simulink model "Simulation_Fahrmodell_v4_straight_line_v2"  (R2023b)
settings: Solver=ode14x  StartTime=0.0  StopTime=500  FixedStep=0.005  RelTol=1e-3
undefined symbols (not defined in the file): bat, cp, cp_Zelle_JpkgK, gb, gb_Gear_Ratio_LUT, gb_Gears_LUT, Ice_derfacLoadDecrease_MAP, Ice_derfacLoadIncrease_MAP, Ice_n_axis, Ice_relLoadMax_CUR_n, Ice_relLoadMax_CUR_val, Ice_rl_axis_norm, P4, P4_DM, pt, seconds, SKO_STREET_CHAL, SKO_WHEEL_TYP_CHAL, slip_pacejka, T_init_degC, Track, TT_sliced, use_turbo_model, v_Fzg_init_kmph, veh, vmax_driver_target_kmh
libraries: nesl_utility x15, fl_lib x9, simulink x4
(part 7 of 7)

== matlab function Simulation_Fahrmodell_v4_straight_line_v2/Vehicle Dynamics Model /Drivetrain/Primary and Secondary Axle Powertrain Selector/MATLAB Function2 ==
  data: Tq_in input; Tq_out output; launchFactor input
function Tq_out = apply_launch_factor(Tq_in, launchFactor)
%#codegen

if Tq_in > 0
    Tq_out = Tq_in * launchFactor;
else
    Tq_out = Tq_in;
end
end

== matlab function Simulation_Fahrmodell_v4_straight_line_v2/Vehicle Dynamics Model /Drivetrain/Axle Load and Torque Distribution /Berechnung Achslastverteilung abh. Fahrzeugeigenschaften (Haken Abs. 11)/MATLAB Function ==
  data: u input; y output
function y = cosd(u)

y = cosd(u);

== matlab function Simulation_Fahrmodell_v4_straight_line_v2/Vehicle Dynamics Model /Drivetrain/Axle Load and Torque Distribution /Berechnung Achslastverteilung abh. Fahrzeugeigenschaften (Haken Abs. 11)/MATLAB Function1 ==
  data: u input; y output
function y = sind(u)

y = sind(u);

== matlab function Simulation_Fahrmodell_v4_straight_line_v2/Vehicle Dynamics Model /Drivetrain/Operating Strategy 1.1/Axle Torque Split/MATLAB Function1 ==
  data: P4_deactivate output; Torque_ICE_Axle_percent output; SOC input; cfg_P4 input; EV input; MainAxle_TorqueSplit_int input; Torque_P4_Axle_percent output
function [P4_deactivate, Torque_ICE_Axle_percent, Torque_P4_Axle_percent]...
        = TorqueSplit(SOC, cfg_P4, EV, MainAxle_TorqueSplit_int)

    % State memory for hysteresis (Lockout flag)
    persistent p4_low_soc_lockout
    if isempty(p4_low_soc_lockout)
        p4_low_soc_lockout = false; 
    end

    % Default: ICE takes all torque, P4 takes none
    Torque_ICE_Axle_percent = 1;
    Torque_P4_Axle_percent = 0;
    P4_deactivate = 0;

    if EV == 1
        P4_split = 1 - MainAxle_TorqueSplit_int;
        Torque_P4_Axle_percent = P4_split;
        Torque_ICE_Axle_percent = 1 - P4_split;
        
    elseif cfg_P4 == 1
        % User-defined P4 split (Main axle = ICE)
        P4_split = 1 - MainAxle_TorqueSplit_int;

        % --- HYSTERESIS LOGIC START ---
        % 1. Determine Lockout State
        if SOC < 0.20
            p4_low_soc_lockout = true;       % Drop below 20%: Lock P4
        elseif SOC >= 0.25
            p4_low_soc_lockout = false;      % Rise above 25%: Unlock P4
        end

        % 2. Apply Limits based on State & SOC
        if p4_low_soc_lockout
            P4_limit = 0;                    % Locked state: 0 torque
        elseif SOC < 0.5
            P4_limit = 0.20;                 % Unlocked but low SOC: Limited torque
        else
            P4_limit = P4_split;             % Healthy SOC: No restriction
        end
        % --- HYSTERESIS LOGIC END ---

        % Apply restriction only if user-defined split exceeds limit
        P4_split = min(P4_split, P4_limit);

        if P4_split == 0
            P4_deactivate = 1;
        else
            P4_deactivate = 0;
        end

        % Assign outputs
        Torque_P4_Axle_percent = P4_split;
        Torque_ICE_Axle_percent = 1 - P4_split;
    end
end

== matlab function Simulation_Fahrmodell_v4_straight_line_v2/Vehicle Dynamics Model /Drivetrain/Operating Strategy 1.1/EM Torque Distributor ==
  data: tq_wheel_EL_des input; tq_wheel_P0_des output; tq_wheel_P2_des output; tq_wheel_P3_des output; Pwr_P0_max_kW input; Pwr_P2_max_kW input; Pwr_P3_max_kW input; cfg_P0 input; cfg_P2 input; cfg_P3 input
function [tq_wheel_P0_des, tq_wheel_P2_des, tq_wheel_P3_des] = ...
    TorqueSplit(tq_wheel_EL_des, Pwr_P0_max_kW, Pwr_P2_max_kW, Pwr_P3_max_kW, ...
                cfg_P0, cfg_P2, cfg_P3)

    % Apply configuration: if cfg = 0, power = 0 (machine disabled)
    P0_active = Pwr_P0_max_kW * cfg_P0;
    P2_active = Pwr_P2_max_kW * cfg_P2;
    P3_active = Pwr_P3_max_kW * cfg_P3;
    
    % Total available power from active machines
    totalPwr = P0_active + P2_active + P3_active;

    % Avoid division by zero (no machine active)
    if totalPwr == 0
        tq_wheel_P0_des = 0;
        tq_wheel_P2_des = 0;
        tq_wheel_P3_des = 0;
        return
    end

    % Ratios based only on active machines
    ratio_P0 = P0_active / totalPwr;
    ratio_P2 = P2_active / totalPwr;
    ratio_P3 = P3_active / totalPwr;

    % Torque split
    tq_wheel_P0_des = ratio_P0 * tq_wheel_EL_des;
    tq_wheel_P2_des = ratio_P2 * tq_wheel_EL_des;
    tq_wheel_P3_des = ratio_P3 * tq_wheel_EL_des;

end

== matlab function Simulation_Fahrmodell_v4_straight_line_v2/Vehicle Dynamics Model /Drivetrain/Operating Strategy 1.1/EMs Priority (Ep)/MATLAB Function ==
  data: tq_ICE_in input; tq_ICE_out output; tq_Elec_in input; SOC input; tq_Elec_out output
function [tq_ICE_out, tq_Elec_out] = TorqueReallocation(tq_ICE_in, tq_Elec_in, SOC)

    % -------------------------------------------------------------
    % HYSTERESIS STATE MEMORY
    % -------------------------------------------------------------
    persistent elec_blocked
    if isempty(elec_blocked)
        elec_blocked = false; % Default: Electric enabled
    end

    % Thresholds
    SOC_Limit = 20;               % Cutoff limit (from your Green block)
    Recovery_Threshold = 25;      % Limit + 5% Hysteresis

    % -------------------------------------------------------------
    % UPDATE STATE (The "Delay Thing")
    % -------------------------------------------------------------
    if SOC < SOC_Limit
        elec_blocked = true;      % SOC dropped too low -> Block Elec
    elseif SOC >= Recovery_Threshold
        elec_blocked = false;     % SOC recovered enough -> Restore Elec
    end
    % Note: If SOC is between 20 and 25, 'elec_blocked' keeps its previous value

    % -------------------------------------------------------------
    % TORQUE LOGIC (From your Diagram)
    % -------------------------------------------------------------
    if elec_blocked
        % LOGIC: SOC is Low (Switch F position)
        % Electric is zeroed.
        % Electric demand is shifted (added) to ICE to compensate.
        tq_Elec_out = 0;
        tq_ICE_out  = tq_ICE_in + tq_Elec_in;
        
    else
        % LOGIC: SOC is Healthy (Switch T position)
        % Inputs pass through unchanged.
        tq_Elec_out = tq_Elec_in;
        tq_ICE_out  = tq_ICE_in;
    end

end

== matlab function Simulation_Fahrmodell_v4_straight_line_v2/Vehicle Dynamics Model /Drivetrain/Primary and Secondary Axle Powertrain Selector/Primary Axle Powertrain Selector/Electric Drive/Variant Subsystem/EV Dual Motor/Battery and Operating Strategy Limitation (Drive)/Discharge Limit/MATLAB Function ==
  settings: updateMethod=DISCRETE
  data: Torque_In input; SOC input; Torque_Out output; Discharge_Limit input
function Torque_Out = fcn(Torque_In, SOC, Discharge_Limit)

% -------------------------------------------------------------
% Corrected SOC Hysteresis Logic
% -------------------------------------------------------------
% If SOC < Discharge_Limit → torque blocked
% Torque stays blocked until SOC >= Discharge_Limit + 10
% -------------------------------------------------------------

persistent torque_blocked

if isempty(torque_blocked)
    torque_blocked = false;   % Start with torque allowed
end

% Hysteresis threshold
Recovery_Threshold = Discharge_Limit + 5;

% --- BLOCKING CONDITION --------------------------------------
if SOC < Discharge_Limit
    torque_blocked = true;
end

% --- RECOVERY CONDITION --------------------------------------
if torque_blocked
    if SOC >= Recovery_Threshold
        torque_blocked = false;   % SOC recovered enough
    else
        Torque_Out = 0;           % Still blocked
        return
    end
end

% --- NORMAL OPERATION ----------------------------------------
Torque_Out = Torque_In;

end

== matlab function Simulation_Fahrmodell_v4_straight_line_v2/Vehicle Dynamics Model /Drivetrain/Primary and Secondary Axle Powertrain Selector/Primary Axle Powertrain Selector/Electric Drive/Variant Subsystem/EV Dual Motor/Battery and Operating Strategy Limitation (Drive) /Discharge Limit1/MATLAB Function ==
  settings: updateMethod=DISCRETE
  data: Torque_In input; SOC input; Torque_Out output; Discharge_Limit input
function Torque_Out = fcn(Torque_In, SOC, Discharge_Limit)

% -------------------------------------------------------------
% Corrected SOC Hysteresis Logic
% -------------------------------------------------------------
% If SOC < Discharge_Limit → torque blocked
% Torque stays blocked until SOC >= Discharge_Limit + 10
% -------------------------------------------------------------

persistent torque_blocked

if isempty(torque_blocked)
    torque_blocked = false;   % Start with torque allowed
end

% Hysteresis threshold
Recovery_Threshold = Discharge_Limit + 5;

% --- BLOCKING CONDITION --------------------------------------
if SOC < Discharge_Limit
    torque_blocked = true;
end

% --- RECOVERY CONDITION --------------------------------------
if torque_blocked
    if SOC >= Recovery_Threshold
        torque_blocked = false;   % SOC recovered enough
    else
        Torque_Out = 0;           % Still blocked
        return
    end
end

% --- NORMAL OPERATION ----------------------------------------
Torque_Out = Torque_In;

end

== matlab function Simulation_Fahrmodell_v4_straight_line_v2/Vehicle Dynamics Model /Drivetrain/Primary and Secondary Axle Powertrain Selector/Primary Axle Powertrain Selector/Electric Drive/Variant Subsystem/EV Single Motor/Battery and Operating Strategy Limitation (Drive)/Discharge Limit/MATLAB Function ==
  settings: updateMethod=DISCRETE
  data: Torque_In input; SOC input; Torque_Out output; Discharge_Limit input
function Torque_Out = fcn(Torque_In, SOC, Discharge_Limit)

% -------------------------------------------------------------
% Corrected SOC Hysteresis Logic
% -------------------------------------------------------------
% If SOC < Discharge_Limit → torque blocked
% Torque stays blocked until SOC >= Discharge_Limit + 10
% -------------------------------------------------------------

persistent torque_blocked

if isempty(torque_blocked)
    torque_blocked = false;   % Start with torque allowed
end

% Hysteresis threshold
Recovery_Threshold = Discharge_Limit + 5;

% --- BLOCKING CONDITION --------------------------------------
if SOC < Discharge_Limit
    torque_blocked = true;
end

% --- RECOVERY CONDITION --------------------------------------
if torque_blocked
    if SOC >= Recovery_Threshold
        torque_blocked = false;   % SOC recovered enough
    else
        Torque_Out = 0;           % Still blocked
        return
    end
end

% --- NORMAL OPERATION ----------------------------------------
Torque_Out = Torque_In;

end

== matlab function Simulation_Fahrmodell_v4_straight_line_v2/Vehicle Dynamics Model /Drivetrain/Primary and Secondary Axle Powertrain Selector/Primary Axle Powertrain Selector/Hybrid Drive/P0/P0 Motor/SubsysteBattery and Operating Strategy Limitation (Drive)m/Discharge Limit/MATLAB Function ==
  settings: updateMethod=DISCRETE
  data: Torque_In input; SOC input; Torque_Out output; Discharge_Limit input
function Torque_Out = fcn(Torque_In, SOC, Discharge_Limit)

% -------------------------------------------------------------
% Corrected SOC Hysteresis Logic
% -------------------------------------------------------------
% If SOC < Discharge_Limit → torque blocked
% Torque stays blocked until SOC >= Discharge_Limit + 10
% -------------------------------------------------------------

persistent torque_blocked

if isempty(torque_blocked)
    torque_blocked = false;   % Start with torque allowed
end

% Hysteresis threshold
Recovery_Threshold = Discharge_Limit + 5;

% --- BLOCKING CONDITION --------------------------------------
if SOC < Discharge_Limit
    torque_blocked = true;
end

% --- RECOVERY CONDITION --------------------------------------
if torque_blocked
    if SOC >= Recovery_Threshold
        torque_blocked = false;   % SOC recovered enough
    else
        Torque_Out = 0;           % Still blocked
        return
    end
end

% --- NORMAL OPERATION ----------------------------------------
Torque_Out = Torque_In;

end

== matlab function Simulation_Fahrmodell_v4_straight_line_v2/Vehicle Dynamics Model /Drivetrain/Primary and Secondary Axle Powertrain Selector/Primary Axle Powertrain Selector/Hybrid Drive/P2/P2 Motor/Battery and Operating Strategy Limitation (Drive)/Discharge Limit/MATLAB Function ==
  settings: updateMethod=DISCRETE
  data: Torque_In input; SOC input; Torque_Out output; Discharge_Limit input
function Torque_Out = fcn(Torque_In, SOC, Discharge_Limit)

% -------------------------------------------------------------
% Corrected SOC Hysteresis Logic
% -------------------------------------------------------------
% If SOC < Discharge_Limit → torque blocked
% Torque stays blocked until SOC >= Discharge_Limit + 10
% -------------------------------------------------------------

persistent torque_blocked

if isempty(torque_blocked)
    torque_blocked = false;   % Start with torque allowed
end

% Hysteresis threshold
Recovery_Threshold = Discharge_Limit + 5;

% --- BLOCKING CONDITION --------------------------------------
if SOC < Discharge_Limit
    torque_blocked = true;
end

% --- RECOVERY CONDITION --------------------------------------
if torque_blocked
    if SOC >= Recovery_Threshold
        torque_blocked = false;   % SOC recovered enough
    else
        Torque_Out = 0;           % Still blocked
        return
    end
end

% --- NORMAL OPERATION ----------------------------------------
Torque_Out = Torque_In;

end

== matlab function Simulation_Fahrmodell_v4_straight_line_v2/Vehicle Dynamics Model /Drivetrain/Primary and Secondary Axle Powertrain Selector/Primary Axle Powertrain Selector/Hybrid Drive/P3/P3 Motor/Battery and Operating Strategy Limitation (Drive)/Discharge Limit/MATLAB Function ==
  settings: updateMethod=DISCRETE
  data: Torque_In input; SOC input; Torque_Out output; Discharge_Limit input
function Torque_Out = fcn(Torque_In, SOC, Discharge_Limit)

% -------------------------------------------------------------
% Corrected SOC Hysteresis Logic
% -------------------------------------------------------------
% If SOC < Discharge_Limit → torque blocked
% Torque stays blocked until SOC >= Discharge_Limit + 10
% -------------------------------------------------------------

persistent torque_blocked

if isempty(torque_blocked)
    torque_blocked = false;   % Start with torque allowed
end

% Hysteresis threshold
Recovery_Threshold = Discharge_Limit + 5;

% --- BLOCKING CONDITION --------------------------------------
if SOC < Discharge_Limit
    torque_blocked = true;
end

% --- RECOVERY CONDITION --------------------------------------
if torque_blocked
    if SOC >= Recovery_Threshold
        torque_blocked = false;   % SOC recovered enough
    else
        Torque_Out = 0;           % Still blocked
        return
    end
end

% --- NORMAL OPERATION ----------------------------------------
Torque_Out = Torque_In;

end

== matlab function Simulation_Fahrmodell_v4_straight_line_v2/Vehicle Dynamics Model /Drivetrain/Axle Load and Torque Distribution /MATLAB Function2 ==
  data: Tq_Primary input; Tq_FrontAxle output; Tq_Secondary input; HM_VA input; AWD input; P4 input; P4_DM input; MainSplit input; Tq_RearAxle output; Tq_grip_FrontMax input; Tq_grip_RearMax input
function [Tq_FrontAxle, Tq_RearAxle] = routeAxleTorqueDynamic( ...
    Tq_Primary, Tq_Secondary, HM_VA, AWD, P4, P4_DM, MainSplit, ...
    Tq_grip_FrontMax, Tq_grip_RearMax)

hasP4 = (P4 == 1) || (P4_DM == 1);

Tq_FrontAxle = 0;
Tq_RearAxle  = 0;

if MainSplit < 0
    MainSplit = 0;
elseif MainSplit > 1
    MainSplit = 1;
end

if AWD == 1 && ~hasP4
    % Mechanisches / variables AWD ohne P4:
    % Gesamtmoment dynamisch nach verfügbarer Traktion verteilen.

    Tq_total = max(Tq_Primary, 0) + max(Tq_Secondary, 0);

    capFront = max(Tq_grip_FrontMax, 0);
    capRear  = max(Tq_grip_RearMax, 0);
    capSum   = capFront + capRear;

    if capSum > 1e-6
        frontShare = capFront / capSum;
    else
        % Fallback: statischer Split
        if HM_VA == 1
            frontShare = MainSplit;
        else
            frontShare = 1 - MainSplit;
        end
    end

    % Optional: nicht zu extreme Splits erlauben
    if frontShare < 0.25
        frontShare = 0.25;
    elseif frontShare > 0.75
        frontShare = 0.75;
    end

    Tq_FrontAxle = frontShare * Tq_total;
    Tq_RearAxle  = (1 - frontShare) * Tq_total;

elseif hasP4
    % P4-Fall: Primary und Secondary bleiben separate Achsantriebe.
    if HM_VA == 1
        Tq_FrontAxle = Tq_Primary;
        Tq_RearAxle  = Tq_Secondary;
    else
        Tq_RearAxle  = Tq_Primary;
        Tq_FrontAxle = Tq_Secondary;
    end

else
    % 2WD-Fall
    if HM_VA == 1
        Tq_FrontAxle = Tq_Primary;
        Tq_RearAxle  = 0;
    else
        Tq_RearAxle  = Tq_Primary;
        Tq_FrontAxle = 0;
    end
end
end

== matlab function Simulation_Fahrmodell_v4_straight_line_v2/Vehicle Dynamics Model /Drivetrain/Primary and Secondary Axle Powertrain Selector/Secondary Axle Powertrain Selector/Auswahl P4, P4_Dual-Motor/P4 // E2 Single Motor/Battery and Operating Strategy Limitation (Drive)/Discharge Limit/MATLAB Function ==
  settings: updateMethod=DISCRETE
  data: Torque_In input; SOC input; Torque_Out output; Discharge_Limit input
function Torque_Out = fcn(Torque_In, SOC, Discharge_Limit)

% -------------------------------------------------------------
% Corrected SOC Hysteresis Logic
% -------------------------------------------------------------
% If SOC < Discharge_Limit → torque blocked
% Torque stays blocked until SOC >= Discharge_Limit + 10
% -------------------------------------------------------------

persistent torque_blocked

if isempty(torque_blocked)
    torque_blocked = false;   % Start with torque allowed
end

% Hysteresis threshold
Recovery_Threshold = Discharge_Limit + 5;

% --- BLOCKING CONDITION --------------------------------------
if SOC < Discharge_Limit
    torque_blocked = true;
end

% --- RECOVERY CONDITION --------------------------------------
if torque_blocked
    if SOC >= Recovery_Threshold
        torque_blocked = false;   % SOC recovered enough
    else
        Torque_Out = 0;           % Still blocked
        return
    end
end

% --- NORMAL OPERATION ----------------------------------------
Torque_Out = Torque_In;

end

== matlab function Simulation_Fahrmodell_v4_straight_line_v2/Vehicle Dynamics Model /Drivetrain/Primary and Secondary Axle Powertrain Selector/Secondary Axle Powertrain Selector/Auswahl P4, P4_Dual-Motor/P4 // E3 // E4 Dual Motor/Battery and Operating Strategy Limitation (Drive) 1/Discharge Limit1/MATLAB Function ==
  settings: updateMethod=DISCRETE
  data: Torque_In input; SOC input; Torque_Out output; Discharge_Limit input
function Torque_Out = fcn(Torque_In, SOC, Discharge_Limit)

% -------------------------------------------------------------
% Corrected SOC Hysteresis Logic
% -------------------------------------------------------------
% If SOC < Discharge_Limit → torque blocked
% Torque stays blocked until SOC >= Discharge_Limit + 10
% -------------------------------------------------------------

persistent torque_blocked

if isempty(torque_blocked)
    torque_blocked = false;   % Start with torque allowed
end

% Hysteresis threshold
Recovery_Threshold = Discharge_Limit + 5;

% --- BLOCKING CONDITION --------------------------------------
if SOC < Discharge_Limit
    torque_blocked = true;
end

% --- RECOVERY CONDITION --------------------------------------
if torque_blocked
    if SOC >= Recovery_Threshold
        torque_blocked = false;   % SOC recovered enough
    else
        Torque_Out = 0;           % Still blocked
        return
    end
end

% --- NORMAL OPERATION ----------------------------------------
Torque_Out = Torque_In;

end

== matlab function Simulation_Fahrmodell_v4_straight_line_v2/Vehicle Dynamics Model /Drivetrain/Primary and Secondary Axle Powertrain Selector/Secondary Axle Powertrain Selector/Auswahl P4, P4_Dual-Motor/P4 // E3 // E4 Dual Motor/Battery and Operating Strategy Limitation (Drive) 2/Discharge Limit/MATLAB Function ==
  settings: updateMethod=DISCRETE
  data: Torque_In input; SOC input; Torque_Out output; Discharge_Limit input
function Torque_Out = fcn(Torque_In, SOC, Discharge_Limit)

% -------------------------------------------------------------
% Corrected SOC Hysteresis Logic
% -------------------------------------------------------------
% If SOC < Discharge_Limit → torque blocked
% Torque stays blocked until SOC >= Discharge_Limit + 10
% -------------------------------------------------------------

persistent torque_blocked

if isempty(torque_blocked)
    torque_blocked = false;   % Start with torque allowed
end

% Hysteresis threshold
Recovery_Threshold = Discharge_Limit + 5;

% --- BLOCKING CONDITION --------------------------------------
if SOC < Discharge_Limit
    torque_blocked = true;
end

% --- RECOVERY CONDITION --------------------------------------
if torque_blocked
    if SOC >= Recovery_Threshold
        torque_blocked = false;   % SOC recovered enough
    else
        Torque_Out = 0;           % Still blocked
        return
    end
end

% --- NORMAL OPERATION ----------------------------------------
Torque_Out = Torque_In;

end

== matlab function Simulation_Fahrmodell_v4_straight_line_v2/Vehicle Dynamics Model /Driving Resistance/Fahrwiderstand/MATLAB Function ==
  data: u input; y output
function y = cosd(u)

y = cosd(u);

== matlab function Simulation_Fahrmodell_v4_straight_line_v2/Vehicle Dynamics Model /Driving Resistance/Fahrwiderstand/MATLAB Function1 ==
  data: u input; y output
function y = sind(u)

y = sind(u);

== matlab function Simulation_Fahrmodell_v4_straight_line_v2/Vehicle Dynamics Model /Driving Resistance/Subsystem/Fahrwiderstand1/MATLAB Function ==
  data: u input; y output
function y = cosd(u)

y = cosd(u);

== matlab function Simulation_Fahrmodell_v4_straight_line_v2/Vehicle Dynamics Model /Driving Resistance/Subsystem/Fahrwiderstand1/MATLAB Function1 ==
  data: u input; y output
function y = sind(u)

y = sind(u);

== matlab function Simulation_Fahrmodell_v4_straight_line_v2/KPIs/MATLAB Function ==
  data: a_mps2 input; stopSim output; dt input
function stopSim = stop_when_accel_low_dt(a_mps2, dt)
%#codegen

a_eps  = 0.05;
T_hold = 2.0;
minTime = 20.0;
maxTime = 120.0;

persistent lowAccelTime simTime

if isempty(lowAccelTime)
    lowAccelTime = 0;
    simTime = 0;
end

simTime = simTime + dt;

if abs(a_mps2) < a_eps
    lowAccelTime = lowAccelTime + dt;
else
    lowAccelTime = 0;
end

stopSim = false;

if simTime >= minTime && lowAccelTime >= T_hold
    stopSim = true;
elseif simTime >= maxTime
    stopSim = true;
end
end

== matlab function Simulation_Fahrmodell_v4_straight_line_v2/Vehicle Dynamics Model /Drivetrain/Axle Load and Torque Distribution 1/Berechnung Achslastverteilung abh. Fahrzeugeigenschaften (Haken Abs. 11)/MATLAB Function ==
  data: u input; y output
function y = cosd(u)

y = cosd(u);

== matlab function Simulation_Fahrmodell_v4_straight_line_v2/Vehicle Dynamics Model /Drivetrain/Axle Load and Torque Distribution 1/Berechnung Achslastverteilung abh. Fahrzeugeigenschaften (Haken Abs. 11)/MATLAB Function1 ==
  data: u input; y output
function y = sind(u)

y = sind(u);

== matlab function Simulation_Fahrmodell_v4_straight_line_v2/Vehicle Dynamics Model /Drivetrain/Axle Load and Torque Distribution 1/Drive Topology Axle Load Distributor /MATLAB Function ==
  data: AWD input; Driven_Wheels_Val output; FWD input; Check_P4 input
function Driven_Wheels_Val  = Driven_Wheels_Selector(AWD, FWD, Check_P4)

% Angetriebene Räder
% 1: Allrad
% 2: Hinterradantrieb
% 3: Vorderradantrieb

% AWD:
% 0 = No
% 1 = Yes
%
% Primary_Axle:
% 0 = Rear
% 1 = Front
%
% Check_P4:
% 0 = No P4 (no AWD unless mentioned)
% 1 = P4 present (AWD always)

Driven_Wheels_Val = 0;

if AWD == 0 && Check_P4 == 0

    if FWD == 0
        Driven_Wheels_Val = 2;
    elseif FWD == 1
        Driven_Wheels_Val = 3;
    end

elseif Check_P4 == 1 || AWD == 1
    Driven_Wheels_Val = 1;
end

== matlab function Simulation_Fahrmodell_v4_straight_line_v2/Vehicle Dynamics Model /Drivetrain/Axle Load and Torque Distribution 1/MATLAB Function ==
  data: Tq_Primary input; Tq_FrontAxle output; Tq_Secondary input; HM_VA input; AWD input; P4 input; P4_DM input; MainSplit input; Tq_RearAxle output
function [Tq_FrontAxle, Tq_RearAxle] = routeAxleTorque( ...
    Tq_Primary, Tq_Secondary, HM_VA, AWD, P4, P4_DM, MainSplit)

hasP4 = (P4 == 1) || (P4_DM == 1);

MainSplit = min(max(MainSplit, 0), 1);

if AWD == 1 && ~hasP4
    % Mechanisches AWD: Primary-Antrieb wird auf beide Achsen verteilt
    if HM_VA == 1
        % Primary axle = vorne
        Tq_FrontAxle = MainSplit * Tq_Primary;
        Tq_RearAxle  = (1 - MainSplit) * Tq_Primary;
    else
        % Primary axle = hinten
        Tq_RearAxle  = MainSplit * Tq_Primary;
        Tq_FrontAxle = (1 - MainSplit) * Tq_Primary;
    end

elseif hasP4
    % Bestehende P4/P4_DM-Logik beibehalten
    if HM_VA == 1
        Tq_FrontAxle = Tq_Primary;
        Tq_RearAxle  = Tq_Secondary;
    else
        Tq_RearAxle  = Tq_Primary;
        Tq_FrontAxle = Tq_Secondary;
    end

else
    % 2WD
    if HM_VA == 1
        Tq_FrontAxle = Tq_Primary;
        Tq_RearAxle  = 0;
    else
        Tq_FrontAxle = 0;
        Tq_RearAxle  = Tq_Primary;
    end
end
end

== matlab function Simulation_Fahrmodell_v4_straight_line_v2/Vehicle Dynamics Model /Drivetrain/Axle Load and Torque Distribution /MATLAB Function1 ==
  data: Tq_FrontAxle input; M_VA_Nm_OUT output; Tq_RearAxle input; Tq_grip_FrontMax input; Tq_grip_RearMax input; M_HA_Nm_OUT output
function [M_VA_Nm_OUT, M_HA_Nm_OUT] = finalAxleTorqueLimiter( ...
    Tq_FrontAxle, Tq_RearAxle, Tq_grip_FrontMax, Tq_grip_RearMax)

M_VA_Nm_OUT = min(max(Tq_FrontAxle, 0), max(Tq_grip_FrontMax, 0));
M_HA_Nm_OUT = min(max(Tq_RearAxle,  0), max(Tq_grip_RearMax,  0));

end
